simulink model "boost_converter_closed_current_loop"  (R2016a)
settings: Solver=ode45  StartTime=0.0  StopTime=50e-3  MaxStep=0.1e-6  RelTol=1e-3
values from neighbouring files (symbols this model uses):
  C = 500e-6    (= 0.0005)    [boost_converter_closed_current_and_voltage_loop_sim_parameters.m]    (also in boost_converter_closed_current_loop_sim_parameters.m)
  D = 1-Vg/Vo    (= 0.6)    [boost_converter_closed_current_and_voltage_loop_sim_parameters.m]    (also in boost_converter_closed_current_loop_sim_parameters.m)
  Gci0 = Gciwc/abs(1+wzc/(i*wc))    [boost_converter_closed_current_and_voltage_loop_sim_parameters.m]    (also in boost_converter_closed_current_loop_sim_parameters.m)
  Io = 30    [boost_converter_closed_current_and_voltage_loop_sim_parameters.m]    (also in boost_converter_closed_current_loop_sim_parameters.m)
  L = 150e-6    (= 0.00015)    [boost_converter_closed_current_and_voltage_loop_sim_parameters.m]    (also in boost_converter_closed_current_loop_sim_parameters.m)
  Rs = 1    [boost_converter_closed_current_and_voltage_loop_sim_parameters.m]    (also in boost_converter_closed_current_loop_sim_parameters.m)
  Vg = 200    [boost_converter_closed_current_and_voltage_loop_sim_parameters.m]    (also in boost_converter_closed_current_loop_sim_parameters.m)
  VM = 1    [boost_converter_closed_current_and_voltage_loop_sim_parameters.m]    (also in boost_converter_closed_current_loop_sim_parameters.m)
  wzc = 2*pi*fzc    (= 2513.27412287)    [boost_converter_closed_current_and_voltage_loop_sim_parameters.m]    (also in boost_converter_closed_current_loop_sim_parameters.m)
libraries: simulink x1
settings Model: Creator=Gorkem  LastModifiedBy=Gorkem
settings GRTTargetCC: GeneratePreprocessorConditionals=Use local settings

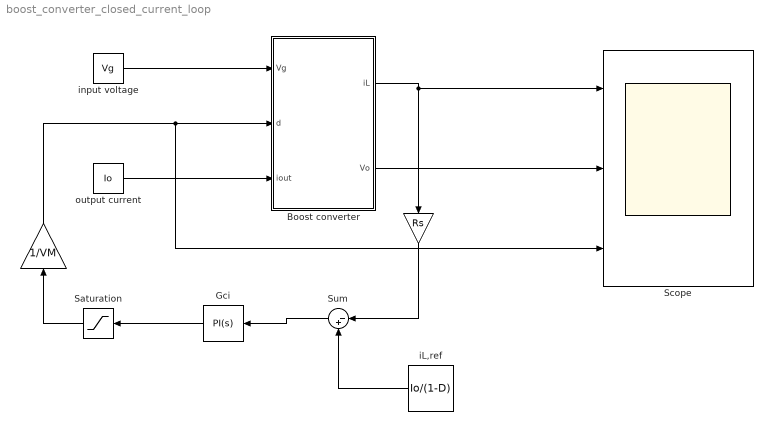
== system boost_converter_closed_current_loop ==
  "  " : Gain  Gain=Rs
  "     " : Gain  Gain=1/VM
  Boost converter : Subsystem
  Gci : simulink/Continuous/PID Controller  Controller=PI  TimeDomain=Continuous-time  SampleTime=-1  IntegratorMethod=Forward Euler  FilterMethod=Forward Euler  Form=Parallel  UseFilter=on  ControllerParametersSource=internal  P=Gci0  I=Gci0*wzc  D=0  N=100  InitialConditionSource=internal  InitialConditionForIntegrator=0  InitialConditionForFilter=0  ExternalReset=none  LimitOutput=off  UpperSaturationLimit=inf  LowerSaturationLimit=-inf  LinearizeAsGain=on  AntiWindupMode=none  Kb=1  TrackingMode=off  Kt=1  PParamMin=[]  PParamMax=[]  IParamMin=[]  IParamMax=[]  DParamMin=[]  DParamMax=[]  NParamMin=[]  NParamMax=[]  KbParamMin=[]  KbParamMax=[]  KtParamMin=[]  KtParamMax=[]  POutMin=[]  POutMax=[]  IOutMin=[]  IOutMax=[]  DOutMin=[]  DOutMax=[]  NOutMin=[]  NOutMax=[]  KbOutMin=[]  KbOutMax=[]  KtOutMin=[]  KtOutMax=[]  IntegratorOutMin=[]  IntegratorOutMax=[]  FilterOutMin=[]  FilterOutMax=[]  SumOutMin=[]  SumOutMax=[]  SumI1OutMin=[]  SumI1OutMax=[]  SumI2OutMin=[]  SumI2OutMax=[]  SumI3OutMin=[]  SumI3OutMax=[]  SumDOutMin=[]  SumDOutMax=[]  SaturationOutMin=[]  SaturationOutMax=[]  IntegratorContinuousStateAttributes=''  IntegratorStateMustResolveToSignalObject=off  IntegratorRTWStateStorageClass=Auto  FilterContinuousStateAttributes=''  FilterStateMustResolveToSignalObject=off  FilterRTWStateStorageClass=Auto  DifferentiatorICPrevScaledInput=0  DifferentiatorOutMin=[]  DifferentiatorOutMax=[]
  Saturation : Saturate  UpperLimit=1  LowerLimit=0
  Scope : Scope  NumInputPorts=3
  Sum : Sum  Inputs=|-+
  iL,ref : Constant  Value=Io/(1-D)
  input voltage : Constant  Value=Vg
  output current : Constant  Value=Io
  wires:
  input voltage/1 -> Boost converter/1(Vg)
  Gci/1 -> Saturation/1
  Boost converter/2(Vo) -> Scope/2
  Boost converter/1(iL) -> "  "/1, Scope/1
  output current/1 -> Boost converter/3(iout)
  iL,ref/1 -> Sum/2
  Sum/1 -> Gci/1
  Saturation/1 -> "     "/1
  "  "/1 -> Sum/1
  "     "/1 -> Scope/3, Boost converter/2(d)

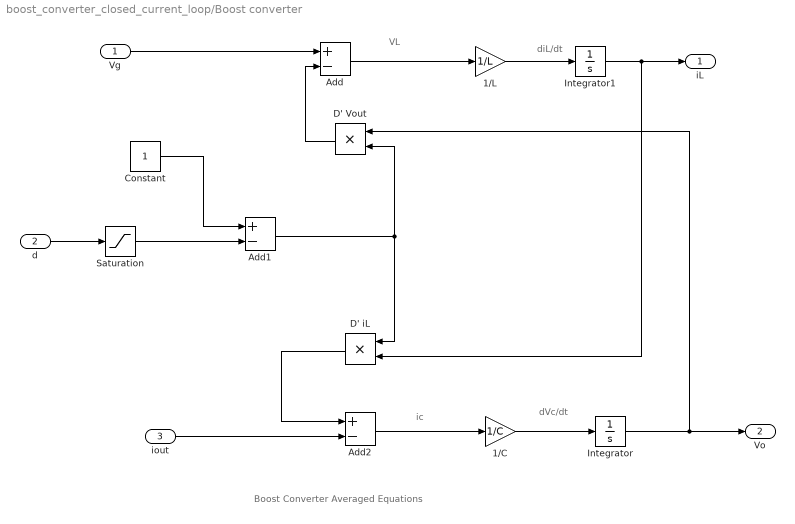
== system boost_converter_closed_current_loop/Boost converter ==
  note: Boost Converter Averaged Equations
  note: dVc/dt
  note: ic
  note: diL/dt
  note: VL
  Vg : Inport
  d : Inport  Port=2
  iout : Inport  Port=3
  1/C : Gain  Gain=1/C
  1/L : Gain  Gain=1/L
  Add : Sum  Inputs=+-
  Add1 : Sum  Inputs=+-
  Add2 : Sum  Inputs=+-
  Constant : Constant
  D' Vout : Product
  D' iL : Product
  Integrator : Integrator
  Integrator1 : Integrator
  Saturation : Saturate  UpperLimit=1  LowerLimit=0
  iL : Outport
  Vo : Outport  Port=2
  wires:
  d/1 -> Saturation/1
  Constant/1 -> Add1/1
  Integrator/1 -> D' Vout/1, Vo/1
  Add1/1 -> D' Vout/2, D' iL/1
  D' Vout/1 -> Add/2
  Vg/1 -> Add/1
  Add/1 -> 1/L/1
  1/L/1 -> Integrator1/1
  Integrator1/1 -> D' iL/2, iL/1
  D' iL/1 -> Add2/1
  iout/1 -> Add2/2
  Add2/1 -> 1/C/1
  1/C/1 -> Integrator/1
  Saturation/1 -> Add1/2
